simulink model "Approx_Multiplier_AMA2_NAB4"  (R2021a)
settings: Solver=FixedStepAuto  StartTime=0.0  StopTime=0.01  FixedStep=0.01  RelTol=1e-3
(part 1 of 3)
settings Model: SimulationMode=accelerator  Creator=PC  LastModifiedBy=PC
settings DataIOCC: ExternalInput=[u]  SaveOutput=off  SignalLogging=off  DSMLogging=off  SaveTime=off  LoggingFileName=Nov_Multiplier.mat
settings HardwareCC: ProdHWDeviceType=AMD->x86-64 (Windows64)

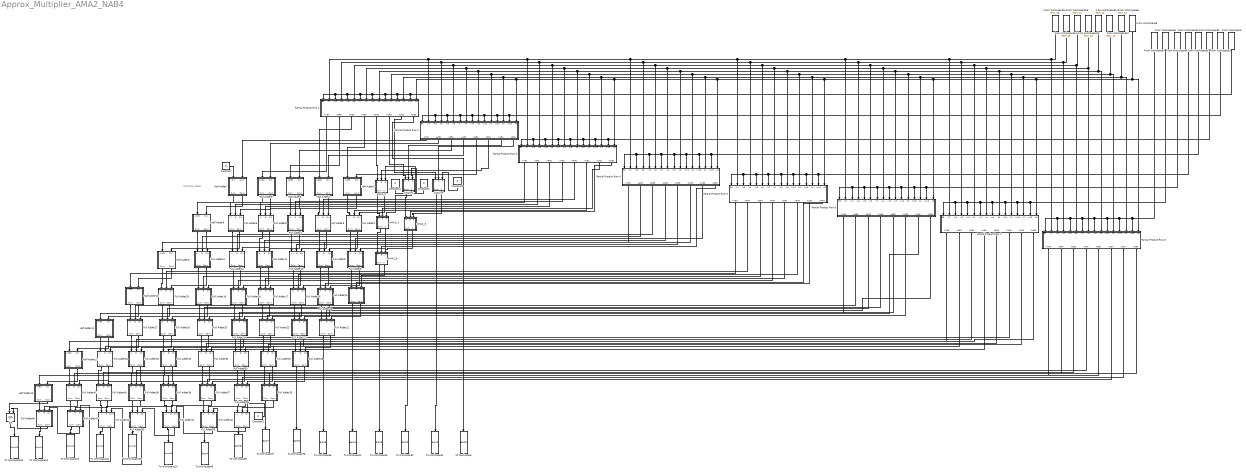
== system Approx_Multiplier_AMA2_NAB4 ==
  note: First Row Done
  AMA2_1 : Subsystem
  AMA2_2 : Subsystem
  AMA2_3 : Subsystem
  AMA2_4 : Subsystem
  AMA2_5 : Subsystem
  AMA2_6 : Subsystem
  Constant{,1..4} (5 alike) : Constant  Value=0
  From Workspace : FromWorkspace  VariableName=Port_1
  From Workspace1 : FromWorkspace  VariableName=Port_2
  From Workspace10 : FromWorkspace  VariableName=Port_11
  From Workspace11 : FromWorkspace  VariableName=Port_12
  From Workspace12 : FromWorkspace  VariableName=Port_13
  From Workspace13 : FromWorkspace  VariableName=Port_14
  From Workspace14 : FromWorkspace  VariableName=Port_15
  From Workspace15 : FromWorkspace  VariableName=Port_16
  From Workspace2 : FromWorkspace  VariableName=Port_3
  From Workspace3 : FromWorkspace  VariableName=Port_4
  From Workspace4 : FromWorkspace  VariableName=Port_5
  From Workspace5 : FromWorkspace  VariableName=Port_6
  From Workspace6 : FromWorkspace  VariableName=Port_7
  From Workspace7 : FromWorkspace  VariableName=Port_8
  From Workspace8 : FromWorkspace  VariableName=Port_9
  From Workspace9 : FromWorkspace  VariableName=Port_10
  Full Adder10 : Subsystem
  Full Adder11 : Subsystem
  Full Adder12 : Subsystem
  Full Adder13 : Subsystem
  Full Adder14 : Subsystem
  Full Adder15 : Subsystem
  Full Adder16 : Subsystem
  Full Adder17 : Subsystem
  Full Adder18 : Subsystem
  Full Adder19 : Subsystem
  Full Adder2 : Subsystem
  Full Adder20 : Subsystem
  Full Adder21 : Subsystem
  Full Adder22 : Subsystem
  Full Adder23 : Subsystem
  Full Adder24 : Subsystem
  Full Adder25 : Subsystem
  Full Adder26 : Subsystem
  Full Adder27 : Subsystem
  Full Adder28 : Subsystem
  Full Adder29 : Subsystem
  Full Adder3 : Subsystem
  Full Adder30 : Subsystem
  Full Adder31 : Subsystem
  Full Adder32 : Subsystem
  Full Adder33 : Subsystem
  Full Adder34 : Subsystem
  Full Adder35 : Subsystem
  Full Adder36 : Subsystem
  Full Adder37 : Subsystem
  Full Adder38 : Subsystem
  Full Adder39 : Subsystem
  Full Adder4 : Subsystem
  Full Adder40 : Subsystem
  Full Adder41 : Subsystem
  Full Adder42 : Subsystem
  Full Adder43 : Subsystem
  Full Adder44 : Subsystem
  Full Adder45 : Subsystem
  Full Adder46 : Subsystem
  Full Adder47 : Subsystem
  Full Adder48 : Subsystem
  Full Adder5 : Subsystem
  Full Adder6 : Subsystem
  Full Adder8 : Subsystem
  Full Adder9 : Subsystem
  Half Adder10 : Subsystem
  Half Adder11 : Subsystem
  Half Adder12 : Subsystem
  Half Adder13 : Subsystem
  Half Adder3 : Subsystem
  Half Adder4 : Subsystem
  Half Adder5 : Subsystem
  Half Adder6 : Subsystem
  Half Adder7 : Subsystem
  Half Adder8 : Subsystem
  Half Adder9 : Subsystem
  OR : Logic  Operator=OR  IconShape=distinctive  AllPortsSameDT=off  OutDataTypeStr=boolean
  Partial Product Row 1 : Subsystem
  Partial Product Row 2 : Subsystem
  Partial Product Row 3 : Subsystem
  Partial Product Row 4 : Subsystem
  Partial Product Row 5 : Subsystem
  Partial Product Row 6 : Subsystem
  Partial Product Row 7 : Subsystem
  Partial Product Row 8 : Subsystem
  To Workspace : ToWorkspace  VariableName=Sum0  SampleTime=0.01
      settings: Save2DSignal=2-D array (concatenate along first dimension)
  To Workspace1 : ToWorkspace  VariableName=Sum1  SampleTime=0.01
      settings: Save2DSignal=2-D array (concatenate along first dimension)
  To Workspace10 : ToWorkspace  VariableName=Sum10  SampleTime=0.01
      settings: Save2DSignal=2-D array (concatenate along first dimension)
  To Workspace11 : ToWorkspace  VariableName=Sum11  SampleTime=0.01
      settings: Save2DSignal=2-D array (concatenate along first dimension)
  To Workspace12 : ToWorkspace  VariableName=Sum12  SampleTime=0.01
      settings: Save2DSignal=2-D array (concatenate along first dimension)
  To Workspace13 : ToWorkspace  VariableName=Sum13  SampleTime=0.01
      settings: Save2DSignal=2-D array (concatenate along first dimension)
  To Workspace14 : ToWorkspace  VariableName=Sum14  SampleTime=0.01
      settings: Save2DSignal=2-D array (concatenate along first dimension)
  To Workspace15 : ToWorkspace  VariableName=Sum15  SampleTime=0.01
      settings: Save2DSignal=2-D array (concatenate along first dimension)
  To Workspace2 : ToWorkspace  VariableName=Sum2  SampleTime=0.01
      settings: Save2DSignal=2-D array (concatenate along first dimension)
  To Workspace3 : ToWorkspace  VariableName=Sum3  SampleTime=0.01
      settings: Save2DSignal=2-D array (concatenate along first dimension)
  To Workspace4 : ToWorkspace  VariableName=Sum4  SampleTime=0.01
      settings: Save2DSignal=2-D array (concatenate along first dimension)
  To Workspace5 : ToWorkspace  VariableName=Sum5  SampleTime=0.01
      settings: Save2DSignal=2-D array (concatenate along first dimension)
  To Workspace6 : ToWorkspace  VariableName=Sum6  SampleTime=0.01
      settings: Save2DSignal=2-D array (concatenate along first dimension)
  To Workspace7 : ToWorkspace  VariableName=Sum7  SampleTime=0.01
      settings: Save2DSignal=2-D array (concatenate along first dimension)
  To Workspace8 : ToWorkspace  VariableName=Sum8  SampleTime=0.01
      settings: Save2DSignal=2-D array (concatenate along first dimension)
  To Workspace9 : ToWorkspace  VariableName=Sum9  SampleTime=0.01
      settings: Save2DSignal=2-D array (concatenate along first dimension)
  wires:
  From Workspace8/1 -> Partial Product Row 8/16(A0), Partial Product Row 7/16(A0), Partial Product Row 6/16(A0), Partial Product Row 4/16(A0), Partial Product Row 3/16(A0), Partial Product Row 1/16(A0), Partial Product Row 2/16(A0), Partial Product Row 5/16(A0)
  From Workspace9/1 -> Partial Product Row 8/14(A1), Partial Product Row 7/14(A1), Partial Product Row 4/14(A1), Partial Product Row 1/14(A1), Partial Product Row 2/14(A1), Partial Product Row 3/14(A1), Partial Product Row 5/14(A1), Partial Product Row 6/14(A1)
  From Workspace10/1 -> Partial Product Row 8/12(A2), Partial Product Row 7/12(A2), Partial Product Row 5/12(A2), Partial Product Row 4/12(A2), Partial Product Row 3/12(A2), Partial Product Row 1/12(A2), Partial Product Row 2/12(A2), Partial Product Row 6/12(A2)
  From Workspace11/1 -> Partial Product Row 8/10(A3), Partial Product Row 6/10(A3), Partial Product Row 4/10(A3), Partial Product Row 3/10(A3), Partial Product Row 1/10(A3), Partial Product Row 2/10(A3), Partial Product Row 5/10(A3), Partial Product Row 7/10(A3)
  From Workspace12/1 -> Partial Product Row 8/8(A4), Partial Product Row 6/8(A4), Partial Product Row 4/8(A4), Partial Product Row 3/8(A4), Partial Product Row 1/8(A4), Partial Product Row 2/8(A4), Partial Product Row 5/8(A4), Partial Product Row 7/8(A4)
  From Workspace13/1 -> Partial Product Row 8/6(A5), Partial Product Row 6/6(A5), Partial Product Row 3/6(A5), Partial Product Row 1/6(A5), Partial Product Row 2/6(A5), Partial Product Row 4/6(A5), Partial Product Row 5/6(A5), Partial Product Row 7/6(A5)
  From Workspace14/1 -> Partial Product Row 8/4(A6), Partial Product Row 7/4(A6), Partial Product Row 6/4(A6), Partial Product Row 5/4(A6), Partial Product Row 4/4(A6), Partial Product Row 3/4(A6), Partial Product Row 1/4(A6), Partial Product Row 2/4(A6)
  From Workspace15/1 -> Partial Product Row 7/2(A7), Partial Product Row 5/2(A7), Partial Product Row 3/2(A7), Partial Product Row 1/2(A7), Partial Product Row 2/2(A7), Partial Product Row 4/2(A7), Partial Product Row 6/2(A7), Partial Product Row 8/2(A7)
  From Workspace/1 -> Partial Product Row 1/3(In3), Partial Product Row 1/1(B0), Partial Product Row 1/5(In5), Partial Product Row 1/7(In7), Partial Product Row 1/9(In9), Partial Product Row 1/11(In11), Partial Product Row 1/13(In13), Partial Product Row 1/15(In15)
  From Workspace1/1 -> Partial Product Row 2/15(In15), Partial Product Row 2/5(In5), Partial Product Row 2/3(In3), Partial Product Row 2/1(B1), Partial Product Row 2/7(In7), Partial Product Row 2/9(In9), Partial Product Row 2/11(In11), Partial Product Row 2/13(In13)
  From Workspace2/1 -> Partial Product Row 3/13(In13), Partial Product Row 3/7(In7), Partial Product Row 3/5(In5), Partial Product Row 3/3(In3), Partial Product Row 3/1(B2), Partial Product Row 3/9(In9), Partial Product Row 3/11(In11), Partial Product Row 3/15(In15)
  From Workspace3/1 -> Partial Product Row 4/13(In13), Partial Product Row 4/11(In11), Partial Product Row 4/9(In9), Partial Product Row 4/5(In5), Partial Product Row 4/3(In3), Partial Product Row 4/1(B3), Partial Product Row 4/7(In7), Partial Product Row 4/15(In15)
  From Workspace4/1 -> Partial Product Row 5/15(In15), Partial Product Row 5/13(In13), Partial Product Row 5/11(In11), Partial Product Row 5/7(In7), Partial Product Row 5/5(In5), Partial Product Row 5/1(B4), Partial Product Row 5/3(In3), Partial Product Row 5/9(In9)
  From Workspace5/1 -> Partial Product Row 6/7(In7), Partial Product Row 6/5(In5), Partial Product Row 6/1(B5), Partial Product Row 6/3(In3), Partial Product Row 6/9(In9), Partial Product Row 6/11(In11), Partial Product Row 6/13(In13), Partial Product Row 6/15(In15)
  From Workspace6/1 -> Partial Product Row 7/13(In13), Partial Product Row 7/7(In7), Partial Product Row 7/5(In5), Partial Product Row 7/1(B6), Partial Product Row 7/3(In3), Partial Product Row 7/9(In9), Partial Product Row 7/11(In11), Partial Product Row 7/15(In15)
  From Workspace7/1 -> Partial Product Row 8/11(In11), Partial Product Row 8/9(In9), Partial Product Row 8/7(In7), Partial Product Row 8/5(In5), Partial Product Row 8/3(In3), Partial Product Row 8/1(B7), Partial Product Row 8/13(In13), Partial Product Row 8/15(In15)
  Partial Product Row 1/7(A1B0) -> AMA2_5/1(A)
  Partial Product Row 2/8(A0B1) -> AMA2_5/2(B)
  Partial Product Row 2/7(A1B1) -> AMA2_1/2(B)
  Partial Product Row 1/6(A2B0) -> AMA2_1/1(A)
  Partial Product Row 1/5(A3B0) -> AMA2_2/1(A)
  Partial Product Row 2/6(A2B1) -> AMA2_2/2(B)
  Partial Product Row 1/4(A4B0) -> Half Adder3/1(A4B0)
  Partial Product Row 2/5(A3B1) -> Half Adder3/2(Cin)
  Partial Product Row 2/4(A4B1) -> Half Adder4/2(Cin)
  Partial Product Row 1/3(A5B0) -> Half Adder4/1(A5B0)
  Partial Product Row 1/2(A6B0) -> Half Adder5/1(A6B0)
  Partial Product Row 2/3(A5B1) -> Half Adder5/2(Cin)
  Partial Product Row 1/1(A7B0) -> Half Adder6/1(A7B0)
  Partial Product Row 2/2(A6B1) -> Half Adder6/2(Cin)
  Constant/1 -> Half Adder7/1(Cin)
  Partial Product Row 2/1(A7B1) -> Half Adder7/2(Cin1)
  AMA2_5/2(Carry) -> AMA2_3/3(Cin)
  AMA2_1/2(Carry) -> AMA2_4/3(Cin)
  AMA2_2/2(Carry) -> Full Adder2/3(Cin)
  Half Adder3/2(Cout) -> Full Adder3/3(Cin)
  Half Adder4/2(Cout) -> Full Adder4/3(Cin)
  Half Adder5/2(Cout) -> Full Adder5/3(Cin)
  Half Adder6/2(Cout) -> Full Adder6/3(Cin)
  Half Adder7/2(Cout) -> Half Adder8/2(Cin)
  AMA2_1/1(Sum) -> AMA2_3/1(A)
  AMA2_2/1(Sum) -> AMA2_4/1(A)
  Half Adder3/1(Sum) -> Full Adder2/1(A)
  Half Adder4/1(Sum) -> Full Adder3/1(A)
  Half Adder5/1(Sum) -> Full Adder4/1(A)
  Half Adder6/1(Sum) -> Full Adder5/1(A)
  Half Adder7/1(Sum) -> Full Adder6/1(A)
  Partial Product Row 3/1(A7B2) -> Half Adder8/1(A7B2)
  Partial Product Row 3/2(A6B2) -> Full Adder6/2(B)
  Partial Product Row 3/3(A5B2) -> Full Adder5/2(B)
  Partial Product Row 3/4(A4B2) -> Full Adder4/2(B)
  Partial Product Row 3/5(A3B2) -> Full Adder3/2(B)
  Partial Product Row 3/6(A2B2) -> Full Adder2/2(B)
  Partial Product Row 3/7(A1B2) -> AMA2_4/2(B)
  Partial Product Row 3/8(A0B2) -> AMA2_3/2(B)
  AMA2_3/2(Carry) -> AMA2_6/3(Cin)
  AMA2_4/2(Carry) -> Full Adder8/3(Cin)
  Full Adder2/2(Carry) -> Full Adder9/3(Cin)
  Full Adder3/2(Carry) -> Full Adder10/3(Cin)
  Full Adder4/2(Carry) -> Full Adder11/3(Cin)
  Full Adder5/2(Carry) -> Full Adder12/3(Cin)
  Full Adder6/2(Carry) -> Full Adder13/3(Cin)
  Half Adder8/2(Cout) -> Half Adder9/2(Cin)
  Half Adder8/1(Sum) -> Full Adder13/1(A)
  Full Adder6/1(Sum) -> Full Adder12/1(A)
  Full Adder5/1(Sum) -> Full Adder11/1(A)
  Full Adder4/1(Sum) -> Full Adder10/1(A)
  Full Adder3/1(Sum) -> Full Adder9/1(A)
  Full Adder2/1(Sum) -> Full Adder8/1(A)
  AMA2_4/1(Sum) -> AMA2_6/1(A)
  Partial Product Row 4/8(A0B3) -> AMA2_6/2(B)
  Partial Product Row 4/7(A1B3) -> Full Adder8/2(B)
  Partial Product Row 4/6(A2B3) -> Full Adder9/2(B)
  Partial Product Row 4/5(A3B3) -> Full Adder10/2(B)
  Partial Product Row 4/4(A4B3) -> Full Adder11/2(B)
  Partial Product Row 4/3(A5B3) -> Full Adder12/2(B)
  Partial Product Row 4/2(A6B3) -> Full Adder13/2(B)
  Partial Product Row 4/1(A7B3) -> Half Adder9/1(A7B2)
  Half Adder9/2(Cout) -> Half Adder10/2(Cin)
  Full Adder13/2(Carry) -> Full Adder20/3(Cin)
  Full Adder12/2(Carry) -> Full Adder19/3(Cin)
  Full Adder11/2(Carry) -> Full Adder18/3(Cin)
  Full Adder10/2(Carry) -> Full Adder17/3(Cin)
  Full Adder9/2(Carry) -> Full Adder16/3(Cin)
  Full Adder8/2(Carry) -> Full Adder15/3(Cin)
  AMA2_6/2(Carry) -> Full Adder14/3(Cin)
  Full Adder8/1(Sum) -> Full Adder14/1(A)
  Full Adder9/1(Sum) -> Full Adder15/1(A)
  Full Adder10/1(Sum) -> Full Adder16/1(A)
  Full Adder11/1(Sum) -> Full Adder17/1(A)
  Full Adder12/1(Sum) -> Full Adder18/1(A)
  Full Adder13/1(Sum) -> Full Adder19/1(A)
  Half Adder9/1(Sum) -> Full Adder20/1(A)
  Partial Product Row 5/8(A0B4) -> Full Adder14/2(B)
  Partial Product Row 5/7(A1B4) -> Full Adder15/2(B)
  Partial Product Row 5/6(A2B4) -> Full Adder16/2(B)
  Partial Product Row 5/5(A3B4) -> Full Adder17/2(B)
  Partial Product Row 5/4(A4B4) -> Full Adder18/2(B)
  Partial Product Row 5/3(A5B4) -> Full Adder19/2(B)
  Partial Product Row 5/2(A6B4) -> Full Adder20/2(B)
  Partial Product Row 5/1(A7B4) -> Half Adder10/1(A7B2)
  Full Adder14/2(Carry) -> Full Adder21/3(Cin)
  Full Adder15/2(Carry) -> Full Adder22/3(Cin)
  Full Adder16/2(Carry) -> Full Adder23/3(Cin)
  Full Adder17/2(Carry) -> Full Adder24/3(Cin)
  Full Adder18/2(Carry) -> Full Adder25/3(Cin)
  Full Adder19/2(Carry) -> Full Adder26/3(Cin)
  Full Adder20/2(Carry) -> Full Adder27/3(Cin)
  Half Adder10/2(Cout) -> Half Adder11/2(Cin)
  Full Adder21/2(Carry) -> Full Adder28/3(Cin)
  Full Adder22/2(Carry) -> Full Adder29/3(Cin)
  Full Adder23/2(Carry) -> Full Adder30/3(Cin)
  Full Adder24/2(Carry) -> Full Adder31/3(Cin)
  Full Adder25/2(Carry) -> Full Adder32/3(Cin)
  Full Adder26/2(Carry) -> Full Adder33/3(Cin)
  Full Adder27/2(Carry) -> Full Adder34/3(Cin)
  Half Adder11/2(Cout) -> Half Adder12/2(Cin)
  Full Adder28/2(Carry) -> Full Adder35/3(Cin)
  Full Adder29/2(Carry) -> Full Adder36/3(Cin)
  Full Adder30/2(Carry) -> Full Adder37/3(Cin)
  Full Adder31/2(Carry) -> Full Adder38/3(Cin)
  Full Adder32/2(Carry) -> Full Adder39/3(Cin)
  Full Adder33/2(Carry) -> Full Adder40/3(Cin)
  Full Adder34/2(Carry) -> Full Adder41/3(Cin)
  Half Adder12/2(Cout) -> Half Adder13/2(Cin)
  Full Adder15/1(Sum) -> Full Adder21/1(A)
  Full Adder16/1(Sum) -> Full Adder22/1(A)
  Full Adder17/1(Sum) -> Full Adder23/1(A)
  Full Adder18/1(Sum) -> Full Adder24/1(A)
  Full Adder19/1(Sum) -> Full Adder25/1(A)
  Full Adder20/1(Sum) -> Full Adder26/1(A)
  Half Adder10/1(Sum) -> Full Adder27/1(A)
  Full Adder22/1(Sum) -> Full Adder28/1(A)
  Full Adder23/1(Sum) -> Full Adder29/1(A)
  Full Adder24/1(Sum) -> Full Adder30/1(A)
  Full Adder25/1(Sum) -> Full Adder31/1(A)
  Full Adder26/1(Sum) -> Full Adder32/1(A)
  Full Adder27/1(Sum) -> Full Adder33/1(A)
  Half Adder11/1(Sum) -> Full Adder34/1(A)
  Full Adder29/1(Sum) -> Full Adder35/1(A)
  Full Adder30/1(Sum) -> Full Adder36/1(A)
  Full Adder31/1(Sum) -> Full Adder37/1(A)
  Full Adder32/1(Sum) -> Full Adder38/1(A)
  Full Adder33/1(Sum) -> Full Adder39/1(A)
  Full Adder34/1(Sum) -> Full Adder40/1(A)
  Half Adder12/1(Sum) -> Full Adder41/1(A)
  Partial Product Row 6/8(A0B5) -> Full Adder21/2(B)
  Partial Product Row 6/7(A1B5) -> Full Adder22/2(B)
  Partial Product Row 6/6(A2B5) -> Full Adder23/2(B)
  Partial Product Row 6/5(A3B5) -> Full Adder24/2(B)
  Partial Product Row 6/4(A4B5) -> Full Adder25/2(B)
  Partial Product Row 6/3(A5B5) -> Full Adder26/2(B)
  Partial Product Row 6/2(A6B5) -> Full Adder27/2(B)
  Partial Product Row 6/1(A7B5) -> Half Adder11/1(A7B2)
  Partial Product Row 7/8(A0B6) -> Full Adder28/2(B)
  Partial Product Row 7/7(A1B6) -> Full Adder29/2(B)
  Partial Product Row 7/6(A2B6) -> Full Adder30/2(B)
  Partial Product Row 7/5(A3B6) -> Full Adder31/2(B)
  Partial Product Row 7/4(A4B6) -> Full Adder32/2(B)
  Partial Product Row 7/3(A5B6) -> Full Adder33/2(B)
  Partial Product Row 7/2(A6B6) -> Full Adder34/2(B)
  Partial Product Row 7/1(A7B6) -> Half Adder12/1(A7B2)
  Partial Product Row 8/8(A0B7) -> Full Adder35/2(B)
  Partial Product Row 8/7(A1B7) -> Full Adder36/2(B)
  Partial Product Row 8/6(A2B7) -> Full Adder37/2(B)
  Partial Product Row 8/5(A3B7) -> Full Adder38/2(B)
  Partial Product Row 8/4(A4B7) -> Full Adder39/2(B)
  Partial Product Row 8/3(A5B7) -> Full Adder40/2(B)
  Partial Product Row 8/2(A6B7) -> Full Adder41/2(B)
  Partial Product Row 8/1(A7B7) -> Half Adder13/1(A7B2)
  Full Adder21/1(Sum) -> To Workspace5/1
  Full Adder14/1(Sum) -> To Workspace4/1
  AMA2_6/1(Sum) -> To Workspace3/1
  AMA2_3/1(Sum) -> To Workspace2/1
  AMA2_5/1(Sum) -> To Workspace1/1
  Partial Product Row 1/8(A0B0) -> To Workspace/1
  Full Adder28/1(Sum) -> To Workspace6/1
  Full Adder35/1(Sum) -> To Workspace7/1
  Full Adder42/1(Sum) -> To Workspace8/1
  Full Adder36/1(Sum) -> Full Adder42/1(A)
  Full Adder43/1(Sum) -> To Workspace9/1
  Full Adder42/2(Carry) -> Full Adder43/3(Cin)
  Full Adder37/1(Sum) -> Full Adder43/1(A)
  Full Adder44/1(Sum) -> To Workspace10/1
  Full Adder43/2(Carry) -> Full Adder44/3(Cin1)
  Full Adder38/1(Sum) -> Full Adder44/1(A)
  Full Adder45/1(Sum) -> To Workspace11/1
  Full Adder44/2(Carry) -> Full Adder45/3(Cin)
  Full Adder39/1(Sum) -> Full Adder45/1(A)
  Full Adder45/2(Carry) -> Full Adder46/3(Cin1)
  Full Adder40/1(Sum) -> Full Adder46/1(A)
  Full Adder47/1(Sum) -> To Workspace13/1
  Full Adder46/1(Sum) -> To Workspace12/1
  Full Adder46/2(Carry) -> Full Adder47/3(Cin)
  Full Adder41/1(Sum) -> Full Adder47/1(A)
  Full Adder48/1(Sum) -> To Workspace14/1
  Full Adder47/2(Carry) -> Full Adder48/3(Cin)
  Half Adder13/1(Sum) -> Full Adder48/1(A)
  Full Adder35/2(Carry) -> Full Adder42/2(B)
  Constant1/1 -> Full Adder42/3(Cin)
  Full Adder36/2(Carry) -> Full Adder43/2(B)
  Full Adder37/2(Carry) -> Full Adder44/2(B)
  Full Adder38/2(Carry) -> Full Adder45/2(B)
  Full Adder39/2(Carry) -> Full Adder46/2(B)
  Full Adder40/2(Carry) -> Full Adder47/2(B)
  Full Adder41/2(Carry) -> Full Adder48/2(B)
  Full Adder48/2(Carry) -> OR/2
  Half Adder13/2(Cout) -> OR/1
  OR/1 -> To Workspace15/1
  Constant3/1 -> AMA2_5/3(Cin)
  Constant2/1 -> AMA2_1/3(Cin)
  Constant4/1 -> AMA2_2/3(Cin)

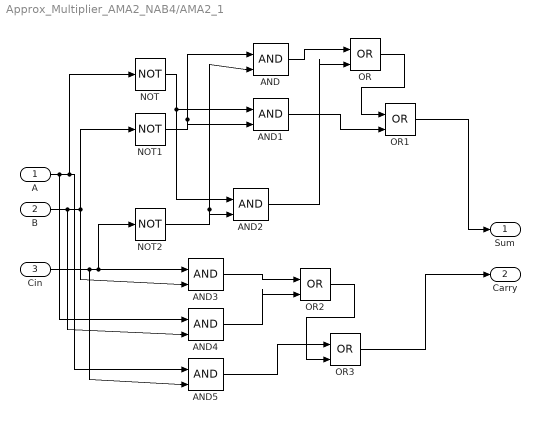
== system Approx_Multiplier_AMA2_NAB4/AMA2_1 ==
  A : Inport
  B : Inport  Port=2
  Cin : Inport  Port=3
  AND{,1..5} (6 alike) : Logic  IconShape=distinctive  AllPortsSameDT=off  OutDataTypeStr=boolean
  NOT : Logic  Operator=NOT  IconShape=distinctive  AllPortsSameDT=off  OutDataTypeStr=boolean
  NOT1 : Logic  Operator=NOT  IconShape=distinctive  AllPortsSameDT=off  OutDataTypeStr=boolean
  NOT2 : Logic  Operator=NOT  IconShape=distinctive  AllPortsSameDT=off  OutDataTypeStr=boolean
  OR{,1..3} (4 alike) : Logic  Operator=OR  IconShape=distinctive  AllPortsSameDT=off  OutDataTypeStr=boolean
  Sum : Outport
  Carry : Outport  Port=2
  wires:
  A/1 -> AND4/1, AND5/1, NOT/1
  B/1 -> AND4/2, AND3/2, NOT1/1
  Cin/1 -> AND5/2, AND3/1, NOT2/1
  NOT2/1 -> AND2/2, AND/2
  NOT1/1 -> AND1/2, AND/1
  NOT/1 -> AND2/1, AND1/1
  AND2/1 -> OR/2
  AND/1 -> OR/1
  OR/1 -> OR1/1
  AND1/1 -> OR1/2
  OR1/1 -> Sum/1
  AND3/1 -> OR2/1
  AND4/1 -> OR2/2
  AND5/1 -> OR3/1
  OR2/1 -> OR3/2
  OR3/1 -> Carry/1

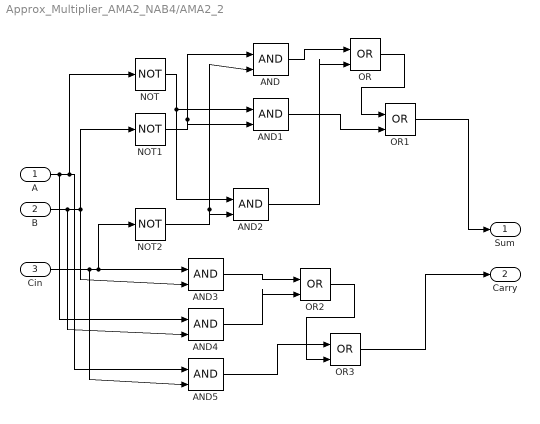
== system Approx_Multiplier_AMA2_NAB4/AMA2_2 ==
  A : Inport
  B : Inport  Port=2
  Cin : Inport  Port=3
  AND{,1..5} (6 alike) : Logic  IconShape=distinctive  AllPortsSameDT=off  OutDataTypeStr=boolean
  NOT : Logic  Operator=NOT  IconShape=distinctive  AllPortsSameDT=off  OutDataTypeStr=boolean
  NOT1 : Logic  Operator=NOT  IconShape=distinctive  AllPortsSameDT=off  OutDataTypeStr=boolean
  NOT2 : Logic  Operator=NOT  IconShape=distinctive  AllPortsSameDT=off  OutDataTypeStr=boolean
  OR{,1..3} (4 alike) : Logic  Operator=OR  IconShape=distinctive  AllPortsSameDT=off  OutDataTypeStr=boolean
  Sum : Outport
  Carry : Outport  Port=2
  wires:
  A/1 -> AND4/1, AND5/1, NOT/1
  B/1 -> AND4/2, AND3/2, NOT1/1
  Cin/1 -> AND5/2, AND3/1, NOT2/1
  NOT2/1 -> AND2/2, AND/2
  NOT1/1 -> AND1/2, AND/1
  NOT/1 -> AND2/1, AND1/1
  AND2/1 -> OR/2
  AND/1 -> OR/1
  OR/1 -> OR1/1
  AND1/1 -> OR1/2
  OR1/1 -> Sum/1
  AND3/1 -> OR2/1
  AND4/1 -> OR2/2
  AND5/1 -> OR3/1
  OR2/1 -> OR3/2
  OR3/1 -> Carry/1

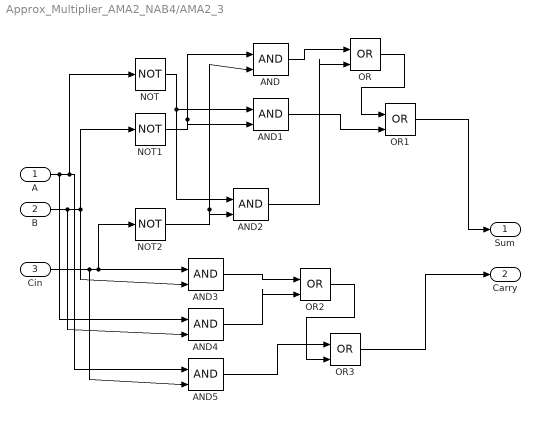
== system Approx_Multiplier_AMA2_NAB4/AMA2_3 ==
  A : Inport
  B : Inport  Port=2
  Cin : Inport  Port=3
  AND{,1..5} (6 alike) : Logic  IconShape=distinctive  AllPortsSameDT=off  OutDataTypeStr=boolean
  NOT : Logic  Operator=NOT  IconShape=distinctive  AllPortsSameDT=off  OutDataTypeStr=boolean
  NOT1 : Logic  Operator=NOT  IconShape=distinctive  AllPortsSameDT=off  OutDataTypeStr=boolean
  NOT2 : Logic  Operator=NOT  IconShape=distinctive  AllPortsSameDT=off  OutDataTypeStr=boolean
  OR{,1..3} (4 alike) : Logic  Operator=OR  IconShape=distinctive  AllPortsSameDT=off  OutDataTypeStr=boolean
  Sum : Outport
  Carry : Outport  Port=2
  wires:
  A/1 -> AND4/1, AND5/1, NOT/1
  B/1 -> AND4/2, AND3/2, NOT1/1
  Cin/1 -> AND5/2, AND3/1, NOT2/1
  NOT2/1 -> AND2/2, AND/2
  NOT1/1 -> AND1/2, AND/1
  NOT/1 -> AND2/1, AND1/1
  AND2/1 -> OR/2
  AND/1 -> OR/1
  OR/1 -> OR1/1
  AND1/1 -> OR1/2
  OR1/1 -> Sum/1
  AND3/1 -> OR2/1
  AND4/1 -> OR2/2
  AND5/1 -> OR3/1
  OR2/1 -> OR3/2
  OR3/1 -> Carry/1

== system Approx_Multiplier_AMA2_NAB4/AMA2_4 ==
  A : Inport
  B : Inport  Port=2
  Cin : Inport  Port=3
  AND{,1..5} (6 alike) : Logic  IconShape=distinctive  AllPortsSameDT=off  OutDataTypeStr=boolean
  NOT : Logic  Operator=NOT  IconShape=distinctive  AllPortsSameDT=off  OutDataTypeStr=boolean
  NOT1 : Logic  Operator=NOT  IconShape=distinctive  AllPortsSameDT=off  OutDataTypeStr=boolean
  NOT2 : Logic  Operator=NOT  IconShape=distinctive  AllPortsSameDT=off  OutDataTypeStr=boolean
  OR{,1..3} (4 alike) : Logic  Operator=OR  IconShape=distinctive  AllPortsSameDT=off  OutDataTypeStr=boolean
  Sum : Outport
  Carry : Outport  Port=2
  wires:
  A/1 -> AND4/1, AND5/1, NOT/1
  B/1 -> AND4/2, AND3/2, NOT1/1
  Cin/1 -> AND5/2, AND3/1, NOT2/1
  NOT2/1 -> AND2/2, AND/2
  NOT1/1 -> AND1/2, AND/1
  NOT/1 -> AND2/1, AND1/1
  AND2/1 -> OR/2
  AND/1 -> OR/1
  OR/1 -> OR1/1
  AND1/1 -> OR1/2
  OR1/1 -> Sum/1
  AND3/1 -> OR2/1
  AND4/1 -> OR2/2
  AND5/1 -> OR3/1
  OR2/1 -> OR3/2
  OR3/1 -> Carry/1

== system Approx_Multiplier_AMA2_NAB4/AMA2_5 ==
  A : Inport
  B : Inport  Port=2
  Cin : Inport  Port=3
  AND{,1..5} (6 alike) : Logic  IconShape=distinctive  AllPortsSameDT=off  OutDataTypeStr=boolean
  NOT : Logic  Operator=NOT  IconShape=distinctive  AllPortsSameDT=off  OutDataTypeStr=boolean
  NOT1 : Logic  Operator=NOT  IconShape=distinctive  AllPortsSameDT=off  OutDataTypeStr=boolean
  NOT2 : Logic  Operator=NOT  IconShape=distinctive  AllPortsSameDT=off  OutDataTypeStr=boolean
  OR{,1..3} (4 alike) : Logic  Operator=OR  IconShape=distinctive  AllPortsSameDT=off  OutDataTypeStr=boolean
  Sum : Outport
  Carry : Outport  Port=2
  wires:
  A/1 -> AND4/1, AND5/1, NOT/1
  B/1 -> AND4/2, AND3/2, NOT1/1
  Cin/1 -> AND5/2, AND3/1, NOT2/1
  NOT2/1 -> AND2/2, AND/2
  NOT1/1 -> AND1/2, AND/1
  NOT/1 -> AND2/1, AND1/1
  AND2/1 -> OR/2
  AND/1 -> OR/1
  OR/1 -> OR1/1
  AND1/1 -> OR1/2
  OR1/1 -> Sum/1
  AND3/1 -> OR2/1
  AND4/1 -> OR2/2
  AND5/1 -> OR3/1
  OR2/1 -> OR3/2
  OR3/1 -> Carry/1

== system Approx_Multiplier_AMA2_NAB4/AMA2_6 ==
  A : Inport
  B : Inport  Port=2
  Cin : Inport  Port=3
  AND{,1..5} (6 alike) : Logic  IconShape=distinctive  AllPortsSameDT=off  OutDataTypeStr=boolean
  NOT : Logic  Operator=NOT  IconShape=distinctive  AllPortsSameDT=off  OutDataTypeStr=boolean
  NOT1 : Logic  Operator=NOT  IconShape=distinctive  AllPortsSameDT=off  OutDataTypeStr=boolean
  NOT2 : Logic  Operator=NOT  IconShape=distinctive  AllPortsSameDT=off  OutDataTypeStr=boolean
  OR{,1..3} (4 alike) : Logic  Operator=OR  IconShape=distinctive  AllPortsSameDT=off  OutDataTypeStr=boolean
  Sum : Outport
  Carry : Outport  Port=2
  wires:
  A/1 -> AND4/1, AND5/1, NOT/1
  B/1 -> AND4/2, AND3/2, NOT1/1
  Cin/1 -> AND5/2, AND3/1, NOT2/1
  NOT2/1 -> AND2/2, AND/2
  NOT1/1 -> AND1/2, AND/1
  NOT/1 -> AND2/1, AND1/1
  AND2/1 -> OR/2
  AND/1 -> OR/1
  OR/1 -> OR1/1
  AND1/1 -> OR1/2
  OR1/1 -> Sum/1
  AND3/1 -> OR2/1
  AND4/1 -> OR2/2
  AND5/1 -> OR3/1
  OR2/1 -> OR3/2
  OR3/1 -> Carry/1

== system Approx_Multiplier_AMA2_NAB4/Full Adder10 ==
  A : Inport
  B : Inport  Port=2
  Cin : Inport  Port=3
  Half Adder : Subsystem
  Half Adder1 : Subsystem
  Logical Operator : Logic  Operator=OR  AllPortsSameDT=off  OutDataTypeStr=boolean
  Sum : Outport
  Carry : Outport  Port=2
  wires:
  Cin/1 -> Half Adder1/1(In)
  Half Adder1/2(Cout) -> Logical Operator/1
  Half Adder/1(Sum) -> Half Adder1/2(Cin)
  Half Adder1/1(Sum) -> Sum/1
  Half Adder/2(Cout) -> Logical Operator/2
  A/1 -> Half Adder/1(In)
  B/1 -> Half Adder/2(Cin)
  Logical Operator/1 -> Carry/1

== system Approx_Multiplier_AMA2_NAB4/Full Adder11 ==
  A : Inport
  B : Inport  Port=2
  Cin : Inport  Port=3
  Half Adder : Subsystem
  Half Adder1 : Subsystem
  Logical Operator : Logic  Operator=OR  AllPortsSameDT=off  OutDataTypeStr=boolean
  Sum : Outport
  Carry : Outport  Port=2
  wires:
  Cin/1 -> Half Adder1/1(In)
  Half Adder1/2(Cout) -> Logical Operator/1
  Half Adder/1(Sum) -> Half Adder1/2(Cin)
  Half Adder1/1(Sum) -> Sum/1
  Half Adder/2(Cout) -> Logical Operator/2
  A/1 -> Half Adder/1(In)
  B/1 -> Half Adder/2(Cin)
  Logical Operator/1 -> Carry/1

== system Approx_Multiplier_AMA2_NAB4/Full Adder12 ==
  A : Inport
  B : Inport  Port=2
  Cin : Inport  Port=3
  Half Adder : Subsystem
  Half Adder1 : Subsystem
  Logical Operator : Logic  Operator=OR  AllPortsSameDT=off  OutDataTypeStr=boolean
  Sum : Outport
  Carry : Outport  Port=2
  wires:
  Cin/1 -> Half Adder1/1(In)
  Half Adder1/2(Cout) -> Logical Operator/1
  Half Adder/1(Sum) -> Half Adder1/2(Cin)
  Half Adder1/1(Sum) -> Sum/1
  Half Adder/2(Cout) -> Logical Operator/2
  A/1 -> Half Adder/1(In)
  B/1 -> Half Adder/2(Cin)
  Logical Operator/1 -> Carry/1

== system Approx_Multiplier_AMA2_NAB4/Full Adder13 ==
  A : Inport
  B : Inport  Port=2
  Cin : Inport  Port=3
  Half Adder : Subsystem
  Half Adder1 : Subsystem
  Logical Operator : Logic  Operator=OR  AllPortsSameDT=off  OutDataTypeStr=boolean
  Sum : Outport
  Carry : Outport  Port=2
  wires:
  Cin/1 -> Half Adder1/1(In)
  Half Adder1/2(Cout) -> Logical Operator/1
  Half Adder/1(Sum) -> Half Adder1/2(Cin)
  Half Adder1/1(Sum) -> Sum/1
  Half Adder/2(Cout) -> Logical Operator/2
  A/1 -> Half Adder/1(In)
  B/1 -> Half Adder/2(Cin)
  Logical Operator/1 -> Carry/1

== system Approx_Multiplier_AMA2_NAB4/Full Adder14 ==
  A : Inport
  B : Inport  Port=2
  Cin : Inport  Port=3
  Half Adder : Subsystem
  Half Adder1 : Subsystem
  Logical Operator : Logic  Operator=OR  AllPortsSameDT=off  OutDataTypeStr=boolean
  Sum : Outport
  Carry : Outport  Port=2
  wires:
  Cin/1 -> Half Adder1/1(In)
  Half Adder1/2(Cout) -> Logical Operator/1
  Half Adder/1(Sum) -> Half Adder1/2(Cin)
  Half Adder1/1(Sum) -> Sum/1
  Half Adder/2(Cout) -> Logical Operator/2
  A/1 -> Half Adder/1(In)
  B/1 -> Half Adder/2(Cin)
  Logical Operator/1 -> Carry/1

== system Approx_Multiplier_AMA2_NAB4/Full Adder15 ==
  A : Inport
  B : Inport  Port=2
  Cin : Inport  Port=3
  Half Adder : Subsystem
  Half Adder1 : Subsystem
  Logical Operator : Logic  Operator=OR  AllPortsSameDT=off  OutDataTypeStr=boolean
  Sum : Outport
  Carry : Outport  Port=2
  wires:
  Cin/1 -> Half Adder1/1(In)
  Half Adder1/2(Cout) -> Logical Operator/1
  Half Adder/1(Sum) -> Half Adder1/2(Cin)
  Half Adder1/1(Sum) -> Sum/1
  Half Adder/2(Cout) -> Logical Operator/2
  A/1 -> Half Adder/1(In)
  B/1 -> Half Adder/2(Cin)
  Logical Operator/1 -> Carry/1

== system Approx_Multiplier_AMA2_NAB4/Full Adder16 ==
  A : Inport
  B : Inport  Port=2
  Cin : Inport  Port=3
  Half Adder : Subsystem
  Half Adder1 : Subsystem
  Logical Operator : Logic  Operator=OR  AllPortsSameDT=off  OutDataTypeStr=boolean
  Sum : Outport
  Carry : Outport  Port=2
  wires:
  Cin/1 -> Half Adder1/1(In)
  Half Adder1/2(Cout) -> Logical Operator/1
  Half Adder/1(Sum) -> Half Adder1/2(Cin)
  Half Adder1/1(Sum) -> Sum/1
  Half Adder/2(Cout) -> Logical Operator/2
  A/1 -> Half Adder/1(In)
  B/1 -> Half Adder/2(Cin)
  Logical Operator/1 -> Carry/1

== system Approx_Multiplier_AMA2_NAB4/Full Adder17 ==
  A : Inport
  B : Inport  Port=2
  Cin : Inport  Port=3
  Half Adder : Subsystem
  Half Adder1 : Subsystem
  Logical Operator : Logic  Operator=OR  AllPortsSameDT=off  OutDataTypeStr=boolean
  Sum : Outport
  Carry : Outport  Port=2
  wires:
  Cin/1 -> Half Adder1/1(In)
  Half Adder1/2(Cout) -> Logical Operator/1
  Half Adder/1(Sum) -> Half Adder1/2(Cin)
  Half Adder1/1(Sum) -> Sum/1
  Half Adder/2(Cout) -> Logical Operator/2
  A/1 -> Half Adder/1(In)
  B/1 -> Half Adder/2(Cin)
  Logical Operator/1 -> Carry/1

== system Approx_Multiplier_AMA2_NAB4/Full Adder18 ==
  A : Inport
  B : Inport  Port=2
  Cin : Inport  Port=3
  Half Adder : Subsystem
  Half Adder1 : Subsystem
  Logical Operator : Logic  Operator=OR  AllPortsSameDT=off  OutDataTypeStr=boolean
  Sum : Outport
  Carry : Outport  Port=2
  wires:
  Cin/1 -> Half Adder1/1(In)
  Half Adder1/2(Cout) -> Logical Operator/1
  Half Adder/1(Sum) -> Half Adder1/2(Cin)
  Half Adder1/1(Sum) -> Sum/1
  Half Adder/2(Cout) -> Logical Operator/2
  A/1 -> Half Adder/1(In)
  B/1 -> Half Adder/2(Cin)
  Logical Operator/1 -> Carry/1

== system Approx_Multiplier_AMA2_NAB4/Full Adder19 ==
  A : Inport
  B : Inport  Port=2
  Cin : Inport  Port=3
  Half Adder : Subsystem
  Half Adder1 : Subsystem
  Logical Operator : Logic  Operator=OR  AllPortsSameDT=off  OutDataTypeStr=boolean
  Sum : Outport
  Carry : Outport  Port=2
  wires:
  Cin/1 -> Half Adder1/1(In)
  Half Adder1/2(Cout) -> Logical Operator/1
  Half Adder/1(Sum) -> Half Adder1/2(Cin)
  Half Adder1/1(Sum) -> Sum/1
  Half Adder/2(Cout) -> Logical Operator/2
  A/1 -> Half Adder/1(In)
  B/1 -> Half Adder/2(Cin)
  Logical Operator/1 -> Carry/1

== system Approx_Multiplier_AMA2_NAB4/Full Adder2 ==
  A : Inport
  B : Inport  Port=2
  Cin : Inport  Port=3
  Half Adder : Subsystem
  Half Adder1 : Subsystem
  Logical Operator : Logic  Operator=OR  AllPortsSameDT=off  OutDataTypeStr=boolean
  Sum : Outport
  Carry : Outport  Port=2
  wires:
  Cin/1 -> Half Adder1/1(In)
  Half Adder1/2(Cout) -> Logical Operator/1
  Half Adder/1(Sum) -> Half Adder1/2(Cin)
  Half Adder1/1(Sum) -> Sum/1
  Half Adder/2(Cout) -> Logical Operator/2
  A/1 -> Half Adder/1(In)
  B/1 -> Half Adder/2(Cin)
  Logical Operator/1 -> Carry/1

== system Approx_Multiplier_AMA2_NAB4/Full Adder20 ==
  A : Inport
  B : Inport  Port=2
  Cin : Inport  Port=3
  Half Adder : Subsystem
  Half Adder1 : Subsystem
  Logical Operator : Logic  Operator=OR  AllPortsSameDT=off  OutDataTypeStr=boolean
  Sum : Outport
  Carry : Outport  Port=2
  wires:
  Cin/1 -> Half Adder1/1(In)
  Half Adder1/2(Cout) -> Logical Operator/1
  Half Adder/1(Sum) -> Half Adder1/2(Cin)
  Half Adder1/1(Sum) -> Sum/1
  Half Adder/2(Cout) -> Logical Operator/2
  A/1 -> Half Adder/1(In)
  B/1 -> Half Adder/2(Cin)
  Logical Operator/1 -> Carry/1

== system Approx_Multiplier_AMA2_NAB4/Full Adder21 ==
  A : Inport
  B : Inport  Port=2
  Cin : Inport  Port=3
  Half Adder : Subsystem
  Half Adder1 : Subsystem
  Logical Operator : Logic  Operator=OR  AllPortsSameDT=off  OutDataTypeStr=boolean
  Sum : Outport
  Carry : Outport  Port=2
  wires:
  Cin/1 -> Half Adder1/1(In)
  Half Adder1/2(Cout) -> Logical Operator/1
  Half Adder/1(Sum) -> Half Adder1/2(Cin)
  Half Adder1/1(Sum) -> Sum/1
  Half Adder/2(Cout) -> Logical Operator/2
  A/1 -> Half Adder/1(In)
  B/1 -> Half Adder/2(Cin)
  Logical Operator/1 -> Carry/1

== system Approx_Multiplier_AMA2_NAB4/Full Adder22 ==
  A : Inport
  B : Inport  Port=2
  Cin : Inport  Port=3
  Half Adder : Subsystem
  Half Adder1 : Subsystem
  Logical Operator : Logic  Operator=OR  AllPortsSameDT=off  OutDataTypeStr=boolean
  Sum : Outport
  Carry : Outport  Port=2
  wires:
  Cin/1 -> Half Adder1/1(In)
  Half Adder1/2(Cout) -> Logical Operator/1
  Half Adder/1(Sum) -> Half Adder1/2(Cin)
  Half Adder1/1(Sum) -> Sum/1
  Half Adder/2(Cout) -> Logical Operator/2
  A/1 -> Half Adder/1(In)
  B/1 -> Half Adder/2(Cin)
  Logical Operator/1 -> Carry/1

== system Approx_Multiplier_AMA2_NAB4/Full Adder23 ==
  A : Inport
  B : Inport  Port=2
  Cin : Inport  Port=3
  Half Adder : Subsystem
  Half Adder1 : Subsystem
  Logical Operator : Logic  Operator=OR  AllPortsSameDT=off  OutDataTypeStr=boolean
  Sum : Outport
  Carry : Outport  Port=2
  wires:
  Cin/1 -> Half Adder1/1(In)
  Half Adder1/2(Cout) -> Logical Operator/1
  Half Adder/1(Sum) -> Half Adder1/2(Cin)
  Half Adder1/1(Sum) -> Sum/1
  Half Adder/2(Cout) -> Logical Operator/2
  A/1 -> Half Adder/1(In)
  B/1 -> Half Adder/2(Cin)
  Logical Operator/1 -> Carry/1

== system Approx_Multiplier_AMA2_NAB4/Full Adder24 ==
  A : Inport
  B : Inport  Port=2
  Cin : Inport  Port=3
  Half Adder : Subsystem
  Half Adder1 : Subsystem
  Logical Operator : Logic  Operator=OR  AllPortsSameDT=off  OutDataTypeStr=boolean
  Sum : Outport
  Carry : Outport  Port=2
  wires:
  Cin/1 -> Half Adder1/1(In)
  Half Adder1/2(Cout) -> Logical Operator/1
  Half Adder/1(Sum) -> Half Adder1/2(Cin)
  Half Adder1/1(Sum) -> Sum/1
  Half Adder/2(Cout) -> Logical Operator/2
  A/1 -> Half Adder/1(In)
  B/1 -> Half Adder/2(Cin)
  Logical Operator/1 -> Carry/1

== system Approx_Multiplier_AMA2_NAB4/Full Adder25 ==
  A : Inport
  B : Inport  Port=2
  Cin : Inport  Port=3
  Half Adder : Subsystem
  Half Adder1 : Subsystem
  Logical Operator : Logic  Operator=OR  AllPortsSameDT=off  OutDataTypeStr=boolean
  Sum : Outport
  Carry : Outport  Port=2
  wires:
  Cin/1 -> Half Adder1/1(In)
  Half Adder1/2(Cout) -> Logical Operator/1
  Half Adder/1(Sum) -> Half Adder1/2(Cin)
  Half Adder1/1(Sum) -> Sum/1
  Half Adder/2(Cout) -> Logical Operator/2
  A/1 -> Half Adder/1(In)
  B/1 -> Half Adder/2(Cin)
  Logical Operator/1 -> Carry/1

== system Approx_Multiplier_AMA2_NAB4/Full Adder26 ==
  A : Inport
  B : Inport  Port=2
  Cin : Inport  Port=3
  Half Adder : Subsystem
  Half Adder1 : Subsystem
  Logical Operator : Logic  Operator=OR  AllPortsSameDT=off  OutDataTypeStr=boolean
  Sum : Outport
  Carry : Outport  Port=2
  wires:
  Cin/1 -> Half Adder1/1(In)
  Half Adder1/2(Cout) -> Logical Operator/1
  Half Adder/1(Sum) -> Half Adder1/2(Cin)
  Half Adder1/1(Sum) -> Sum/1
  Half Adder/2(Cout) -> Logical Operator/2
  A/1 -> Half Adder/1(In)
  B/1 -> Half Adder/2(Cin)
  Logical Operator/1 -> Carry/1

== system Approx_Multiplier_AMA2_NAB4/Full Adder27 ==
  A : Inport
  B : Inport  Port=2
  Cin : Inport  Port=3
  Half Adder : Subsystem
  Half Adder1 : Subsystem
  Logical Operator : Logic  Operator=OR  AllPortsSameDT=off  OutDataTypeStr=boolean
  Sum : Outport
  Carry : Outport  Port=2
  wires:
  Cin/1 -> Half Adder1/1(In)
  Half Adder1/2(Cout) -> Logical Operator/1
  Half Adder/1(Sum) -> Half Adder1/2(Cin)
  Half Adder1/1(Sum) -> Sum/1
  Half Adder/2(Cout) -> Logical Operator/2
  A/1 -> Half Adder/1(In)
  B/1 -> Half Adder/2(Cin)
  Logical Operator/1 -> Carry/1

== system Approx_Multiplier_AMA2_NAB4/Full Adder28 ==
  A : Inport
  B : Inport  Port=2
  Cin : Inport  Port=3
  Half Adder : Subsystem
  Half Adder1 : Subsystem
  Logical Operator : Logic  Operator=OR  AllPortsSameDT=off  OutDataTypeStr=boolean
  Sum : Outport
  Carry : Outport  Port=2
  wires:
  Cin/1 -> Half Adder1/1(In)
  Half Adder1/2(Cout) -> Logical Operator/1
  Half Adder/1(Sum) -> Half Adder1/2(Cin)
  Half Adder1/1(Sum) -> Sum/1
  Half Adder/2(Cout) -> Logical Operator/2
  A/1 -> Half Adder/1(In)
  B/1 -> Half Adder/2(Cin)
  Logical Operator/1 -> Carry/1

== system Approx_Multiplier_AMA2_NAB4/Full Adder29 ==
  A : Inport
  B : Inport  Port=2
  Cin : Inport  Port=3
  Half Adder : Subsystem
  Half Adder1 : Subsystem
  Logical Operator : Logic  Operator=OR  AllPortsSameDT=off  OutDataTypeStr=boolean
  Sum : Outport
  Carry : Outport  Port=2
  wires:
  Cin/1 -> Half Adder1/1(In)
  Half Adder1/2(Cout) -> Logical Operator/1
  Half Adder/1(Sum) -> Half Adder1/2(Cin)
  Half Adder1/1(Sum) -> Sum/1
  Half Adder/2(Cout) -> Logical Operator/2
  A/1 -> Half Adder/1(In)
  B/1 -> Half Adder/2(Cin)
  Logical Operator/1 -> Carry/1

== system Approx_Multiplier_AMA2_NAB4/Full Adder3 ==
  A : Inport
  B : Inport  Port=2
  Cin : Inport  Port=3
  Half Adder : Subsystem
  Half Adder1 : Subsystem
  Logical Operator : Logic  Operator=OR  AllPortsSameDT=off  OutDataTypeStr=boolean
  Sum : Outport
  Carry : Outport  Port=2
  wires:
  Cin/1 -> Half Adder1/1(In)
  Half Adder1/2(Cout) -> Logical Operator/1
  Half Adder/1(Sum) -> Half Adder1/2(Cin)
  Half Adder1/1(Sum) -> Sum/1
  Half Adder/2(Cout) -> Logical Operator/2
  A/1 -> Half Adder/1(In)
  B/1 -> Half Adder/2(Cin)
  Logical Operator/1 -> Carry/1

== system Approx_Multiplier_AMA2_NAB4/Full Adder30 ==
  A : Inport
  B : Inport  Port=2
  Cin : Inport  Port=3
  Half Adder : Subsystem
  Half Adder1 : Subsystem
  Logical Operator : Logic  Operator=OR  AllPortsSameDT=off  OutDataTypeStr=boolean
  Sum : Outport
  Carry : Outport  Port=2
  wires:
  Cin/1 -> Half Adder1/1(In)
  Half Adder1/2(Cout) -> Logical Operator/1
  Half Adder/1(Sum) -> Half Adder1/2(Cin)
  Half Adder1/1(Sum) -> Sum/1
  Half Adder/2(Cout) -> Logical Operator/2
  A/1 -> Half Adder/1(In)
  B/1 -> Half Adder/2(Cin)
  Logical Operator/1 -> Carry/1

== system Approx_Multiplier_AMA2_NAB4/Full Adder31 ==
  A : Inport
  B : Inport  Port=2
  Cin : Inport  Port=3
  Half Adder : Subsystem
  Half Adder1 : Subsystem
  Logical Operator : Logic  Operator=OR  AllPortsSameDT=off  OutDataTypeStr=boolean
  Sum : Outport
  Carry : Outport  Port=2
  wires:
  Cin/1 -> Half Adder1/1(In)
  Half Adder1/2(Cout) -> Logical Operator/1
  Half Adder/1(Sum) -> Half Adder1/2(Cin)
  Half Adder1/1(Sum) -> Sum/1
  Half Adder/2(Cout) -> Logical Operator/2
  A/1 -> Half Adder/1(In)
  B/1 -> Half Adder/2(Cin)
  Logical Operator/1 -> Carry/1

== system Approx_Multiplier_AMA2_NAB4/Full Adder32 ==
  A : Inport
  B : Inport  Port=2
  Cin : Inport  Port=3
  Half Adder : Subsystem
  Half Adder1 : Subsystem
  Logical Operator : Logic  Operator=OR  AllPortsSameDT=off  OutDataTypeStr=boolean
  Sum : Outport
  Carry : Outport  Port=2
  wires:
  Cin/1 -> Half Adder1/1(In)
  Half Adder1/2(Cout) -> Logical Operator/1
  Half Adder/1(Sum) -> Half Adder1/2(Cin)
  Half Adder1/1(Sum) -> Sum/1
  Half Adder/2(Cout) -> Logical Operator/2
  A/1 -> Half Adder/1(In)
  B/1 -> Half Adder/2(Cin)
  Logical Operator/1 -> Carry/1

== system Approx_Multiplier_AMA2_NAB4/Full Adder33 ==
  A : Inport
  B : Inport  Port=2
  Cin : Inport  Port=3
  Half Adder : Subsystem
  Half Adder1 : Subsystem
  Logical Operator : Logic  Operator=OR  AllPortsSameDT=off  OutDataTypeStr=boolean
  Sum : Outport
  Carry : Outport  Port=2
  wires:
  Cin/1 -> Half Adder1/1(In)
  Half Adder1/2(Cout) -> Logical Operator/1
  Half Adder/1(Sum) -> Half Adder1/2(Cin)
  Half Adder1/1(Sum) -> Sum/1
  Half Adder/2(Cout) -> Logical Operator/2
  A/1 -> Half Adder/1(In)
  B/1 -> Half Adder/2(Cin)
  Logical Operator/1 -> Carry/1

== system Approx_Multiplier_AMA2_NAB4/Full Adder34 ==
  A : Inport
  B : Inport  Port=2
  Cin : Inport  Port=3
  Half Adder : Subsystem
  Half Adder1 : Subsystem
  Logical Operator : Logic  Operator=OR  AllPortsSameDT=off  OutDataTypeStr=boolean
  Sum : Outport
  Carry : Outport  Port=2
  wires:
  Cin/1 -> Half Adder1/1(In)
  Half Adder1/2(Cout) -> Logical Operator/1
  Half Adder/1(Sum) -> Half Adder1/2(Cin)
  Half Adder1/1(Sum) -> Sum/1
  Half Adder/2(Cout) -> Logical Operator/2
  A/1 -> Half Adder/1(In)
  B/1 -> Half Adder/2(Cin)
  Logical Operator/1 -> Carry/1

== system Approx_Multiplier_AMA2_NAB4/Full Adder35 ==
  A : Inport
  B : Inport  Port=2
  Cin : Inport  Port=3
  Half Adder : Subsystem
  Half Adder1 : Subsystem
  Logical Operator : Logic  Operator=OR  AllPortsSameDT=off  OutDataTypeStr=boolean
  Sum : Outport
  Carry : Outport  Port=2
  wires:
  Cin/1 -> Half Adder1/1(In)
  Half Adder1/2(Cout) -> Logical Operator/1
  Half Adder/1(Sum) -> Half Adder1/2(Cin)
  Half Adder1/1(Sum) -> Sum/1
  Half Adder/2(Cout) -> Logical Operator/2
  A/1 -> Half Adder/1(In)
  B/1 -> Half Adder/2(Cin)
  Logical Operator/1 -> Carry/1

== system Approx_Multiplier_AMA2_NAB4/Full Adder36 ==
  A : Inport
  B : Inport  Port=2
  Cin : Inport  Port=3
  Half Adder : Subsystem
  Half Adder1 : Subsystem
  Logical Operator : Logic  Operator=OR  AllPortsSameDT=off  OutDataTypeStr=boolean
  Sum : Outport
  Carry : Outport  Port=2
  wires:
  Cin/1 -> Half Adder1/1(In)
  Half Adder1/2(Cout) -> Logical Operator/1
  Half Adder/1(Sum) -> Half Adder1/2(Cin)
  Half Adder1/1(Sum) -> Sum/1
  Half Adder/2(Cout) -> Logical Operator/2
  A/1 -> Half Adder/1(In)
  B/1 -> Half Adder/2(Cin)
  Logical Operator/1 -> Carry/1

== system Approx_Multiplier_AMA2_NAB4/Full Adder37 ==
  A : Inport
  B : Inport  Port=2
  Cin : Inport  Port=3
  Half Adder : Subsystem
  Half Adder1 : Subsystem
  Logical Operator : Logic  Operator=OR  AllPortsSameDT=off  OutDataTypeStr=boolean
  Sum : Outport
  Carry : Outport  Port=2
  wires:
  Cin/1 -> Half Adder1/1(In)
  Half Adder1/2(Cout) -> Logical Operator/1
  Half Adder/1(Sum) -> Half Adder1/2(Cin)
  Half Adder1/1(Sum) -> Sum/1
  Half Adder/2(Cout) -> Logical Operator/2
  A/1 -> Half Adder/1(In)
  B/1 -> Half Adder/2(Cin)
  Logical Operator/1 -> Carry/1

== system Approx_Multiplier_AMA2_NAB4/Full Adder38 ==
  A : Inport
  B : Inport  Port=2
  Cin : Inport  Port=3
  Half Adder : Subsystem
  Half Adder1 : Subsystem
  Logical Operator : Logic  Operator=OR  AllPortsSameDT=off  OutDataTypeStr=boolean
  Sum : Outport
  Carry : Outport  Port=2
  wires:
  Cin/1 -> Half Adder1/1(In)
  Half Adder1/2(Cout) -> Logical Operator/1
  Half Adder/1(Sum) -> Half Adder1/2(Cin)
  Half Adder1/1(Sum) -> Sum/1
  Half Adder/2(Cout) -> Logical Operator/2
  A/1 -> Half Adder/1(In)
  B/1 -> Half Adder/2(Cin)
  Logical Operator/1 -> Carry/1

== system Approx_Multiplier_AMA2_NAB4/Full Adder39 ==
  A : Inport
  B : Inport  Port=2
  Cin : Inport  Port=3
  Half Adder : Subsystem
  Half Adder1 : Subsystem
  Logical Operator : Logic  Operator=OR  AllPortsSameDT=off  OutDataTypeStr=boolean
  Sum : Outport
  Carry : Outport  Port=2
  wires:
  Cin/1 -> Half Adder1/1(In)
  Half Adder1/2(Cout) -> Logical Operator/1
  Half Adder/1(Sum) -> Half Adder1/2(Cin)
  Half Adder1/1(Sum) -> Sum/1
  Half Adder/2(Cout) -> Logical Operator/2
  A/1 -> Half Adder/1(In)
  B/1 -> Half Adder/2(Cin)
  Logical Operator/1 -> Carry/1

== system Approx_Multiplier_AMA2_NAB4/Full Adder4 ==
  A : Inport
  B : Inport  Port=2
  Cin : Inport  Port=3
  Half Adder : Subsystem
  Half Adder1 : Subsystem
  Logical Operator : Logic  Operator=OR  AllPortsSameDT=off  OutDataTypeStr=boolean
  Sum : Outport
  Carry : Outport  Port=2
  wires:
  Cin/1 -> Half Adder1/1(In)
  Half Adder1/2(Cout) -> Logical Operator/1
  Half Adder/1(Sum) -> Half Adder1/2(Cin)
  Half Adder1/1(Sum) -> Sum/1
  Half Adder/2(Cout) -> Logical Operator/2
  A/1 -> Half Adder/1(In)
  B/1 -> Half Adder/2(Cin)
  Logical Operator/1 -> Carry/1

== system Approx_Multiplier_AMA2_NAB4/Full Adder40 ==
  A : Inport
  B : Inport  Port=2
  Cin : Inport  Port=3
  Half Adder : Subsystem
  Half Adder1 : Subsystem
  Logical Operator : Logic  Operator=OR  AllPortsSameDT=off  OutDataTypeStr=boolean
  Sum : Outport
  Carry : Outport  Port=2
  wires:
  Cin/1 -> Half Adder1/1(In)
  Half Adder1/2(Cout) -> Logical Operator/1
  Half Adder/1(Sum) -> Half Adder1/2(Cin)
  Half Adder1/1(Sum) -> Sum/1
  Half Adder/2(Cout) -> Logical Operator/2
  A/1 -> Half Adder/1(In)
  B/1 -> Half Adder/2(Cin)
  Logical Operator/1 -> Carry/1

== system Approx_Multiplier_AMA2_NAB4/Full Adder41 ==
  A : Inport
  B : Inport  Port=2
  Cin : Inport  Port=3
  Half Adder : Subsystem
  Half Adder1 : Subsystem
  Logical Operator : Logic  Operator=OR  AllPortsSameDT=off  OutDataTypeStr=boolean
  Sum : Outport
  Carry : Outport  Port=2
  wires:
  Cin/1 -> Half Adder1/1(In)
  Half Adder1/2(Cout) -> Logical Operator/1
  Half Adder/1(Sum) -> Half Adder1/2(Cin)
  Half Adder1/1(Sum) -> Sum/1
  Half Adder/2(Cout) -> Logical Operator/2
  A/1 -> Half Adder/1(In)
  B/1 -> Half Adder/2(Cin)
  Logical Operator/1 -> Carry/1

== system Approx_Multiplier_AMA2_NAB4/Full Adder42 ==
  A : Inport
  B : Inport  Port=2
  Cin : Inport  Port=3
  Half Adder : Subsystem
  Half Adder1 : Subsystem
  Logical Operator : Logic  Operator=OR  AllPortsSameDT=off  OutDataTypeStr=boolean
  Sum : Outport
  Carry : Outport  Port=2
  wires:
  Cin/1 -> Half Adder1/1(In)
  Half Adder1/2(Cout) -> Logical Operator/1
  Half Adder/1(Sum) -> Half Adder1/2(Cin)
  Half Adder1/1(Sum) -> Sum/1
  Half Adder/2(Cout) -> Logical Operator/2
  A/1 -> Half Adder/1(In)
  B/1 -> Half Adder/2(Cin)
  Logical Operator/1 -> Carry/1

== system Approx_Multiplier_AMA2_NAB4/Full Adder43 ==
  A : Inport
  B : Inport  Port=2
  Cin : Inport  Port=3
  Half Adder : Subsystem
  Half Adder1 : Subsystem
  Logical Operator : Logic  Operator=OR  AllPortsSameDT=off  OutDataTypeStr=boolean
  Sum : Outport
  Carry : Outport  Port=2
  wires:
  Half Adder1/2(Cout) -> Logical Operator/1
  Half Adder/1(Sum) -> Half Adder1/2(Cin)
  Half Adder1/1(Sum) -> Sum/1
  Half Adder/2(Cout) -> Logical Operator/2
  A/1 -> Half Adder/1(In)
  B/1 -> Half Adder/2(Cin)
  Logical Operator/1 -> Carry/1
  Cin/1 -> Half Adder1/1(In)

== system Approx_Multiplier_AMA2_NAB4/Full Adder44 ==
  A : Inport
  B : Inport  Port=2
  Cin1 : Inport  Port=3
  Half Adder : Subsystem
  Half Adder1 : Subsystem
  Logical Operator : Logic  Operator=OR  AllPortsSameDT=off  OutDataTypeStr=boolean
  Sum : Outport
  Carry : Outport  Port=2
  wires:
  Half Adder1/2(Cout) -> Logical Operator/1
  Half Adder/1(Sum) -> Half Adder1/2(Cin)
  Half Adder1/1(Sum) -> Sum/1
  Half Adder/2(Cout) -> Logical Operator/2
  A/1 -> Half Adder/1(In)
  B/1 -> Half Adder/2(Cin)
  Logical Operator/1 -> Carry/1
  Cin1/1 -> Half Adder1/1(Cin1)

== system Approx_Multiplier_AMA2_NAB4/Full Adder45 ==
  A : Inport
  B : Inport  Port=2
  Cin : Inport  Port=3
  Half Adder : Subsystem
  Half Adder1 : Subsystem
  Logical Operator : Logic  Operator=OR  AllPortsSameDT=off  OutDataTypeStr=boolean
  Sum : Outport
  Carry : Outport  Port=2
  wires:
  Half Adder1/2(Cout) -> Logical Operator/1
  Half Adder/1(Sum) -> Half Adder1/2(Cin)
  Half Adder1/1(Sum) -> Sum/1
  Half Adder/2(Cout) -> Logical Operator/2
  A/1 -> Half Adder/1(In)
  B/1 -> Half Adder/2(Cin)
  Logical Operator/1 -> Carry/1
  Cin/1 -> Half Adder1/1(In)

== system Approx_Multiplier_AMA2_NAB4/Full Adder46 ==
  A : Inport
  B : Inport  Port=2
  Cin1 : Inport  Port=3
  Half Adder : Subsystem
  Half Adder1 : Subsystem
  Logical Operator : Logic  Operator=OR  AllPortsSameDT=off  OutDataTypeStr=boolean
  Sum : Outport
  Carry : Outport  Port=2
  wires:
  Half Adder1/2(Cout) -> Logical Operator/1
  Half Adder/1(Sum) -> Half Adder1/2(Cin)
  Half Adder1/1(Sum) -> Sum/1
  Half Adder/2(Cout) -> Logical Operator/2
  A/1 -> Half Adder/1(In)
  B/1 -> Half Adder/2(Cin)
  Logical Operator/1 -> Carry/1
  Cin1/1 -> Half Adder1/1(Cin1)

== system Approx_Multiplier_AMA2_NAB4/Full Adder47 ==
  A : Inport
  B : Inport  Port=2
  Cin : Inport  Port=3
  Half Adder : Subsystem
  Half Adder1 : Subsystem
  Logical Operator : Logic  Operator=OR  AllPortsSameDT=off  OutDataTypeStr=boolean
  Sum : Outport
  Carry : Outport  Port=2
  wires:
  Half Adder1/2(Cout) -> Logical Operator/1
  Half Adder/1(Sum) -> Half Adder1/2(Cin)
  Half Adder1/1(Sum) -> Sum/1
  Half Adder/2(Cout) -> Logical Operator/2
  A/1 -> Half Adder/1(In)
  B/1 -> Half Adder/2(Cin)
  Logical Operator/1 -> Carry/1
  Cin/1 -> Half Adder1/1(In)

== system Approx_Multiplier_AMA2_NAB4/Full Adder48 ==
  A : Inport
  B : Inport  Port=2
  Cin : Inport  Port=3
  Half Adder : Subsystem
  Half Adder1 : Subsystem
  Logical Operator : Logic  Operator=OR  AllPortsSameDT=off  OutDataTypeStr=boolean
  Sum : Outport
  Carry : Outport  Port=2
  wires:
  Half Adder1/2(Cout) -> Logical Operator/1
  Half Adder/1(Sum) -> Half Adder1/2(Cin)
  Half Adder1/1(Sum) -> Sum/1
  Half Adder/2(Cout) -> Logical Operator/2
  A/1 -> Half Adder/1(In)
  B/1 -> Half Adder/2(Cin)
  Logical Operator/1 -> Carry/1
  Cin/1 -> Half Adder1/1(In)

== system Approx_Multiplier_AMA2_NAB4/Full Adder5 ==
  A : Inport
  B : Inport  Port=2
  Cin : Inport  Port=3
  Half Adder : Subsystem
  Half Adder1 : Subsystem
  Logical Operator : Logic  Operator=OR  AllPortsSameDT=off  OutDataTypeStr=boolean
  Sum : Outport
  Carry : Outport  Port=2
  wires:
  Cin/1 -> Half Adder1/1(In)
  Half Adder1/2(Cout) -> Logical Operator/1
  Half Adder/1(Sum) -> Half Adder1/2(Cin)
  Half Adder1/1(Sum) -> Sum/1
  Half Adder/2(Cout) -> Logical Operator/2
  A/1 -> Half Adder/1(In)
  B/1 -> Half Adder/2(Cin)
  Logical Operator/1 -> Carry/1
